simulink library "component_lib"  (R2023a)
settings: Solver=VariableStepAuto  StartTime=0.0  StopTime=10.0  RelTol=1e-3
undefined symbols (not defined in the file or in its folder): ECCV_r, par, R1234yf_ph, V_nom
libraries: base_lib x258, $bdroot x212, simulink x2, slpidlib x1
(part 1 of 7)
settings Model: Creator=maxjo65  LastModifiedBy=maxjo
settings SolverCC: AlgebraicLoopSolver=TrustRegion
settings OptimizationCC: ReuseModelBlockBuffer=off
settings DebuggingCC: UnconnectedInputMsg=warning  UnconnectedOutputMsg=warning  UnconnectedLineMsg=warning
settings ModelReferenceCC: EnableRefExpFcnMdlSchedulingChecks=on
settings RTWCC: DLArmComputeVersion=19.05

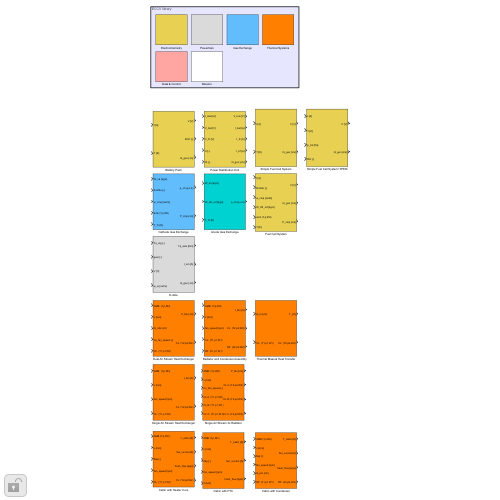
[thumbnail: Simulink's stored preview of the top-level diagram]
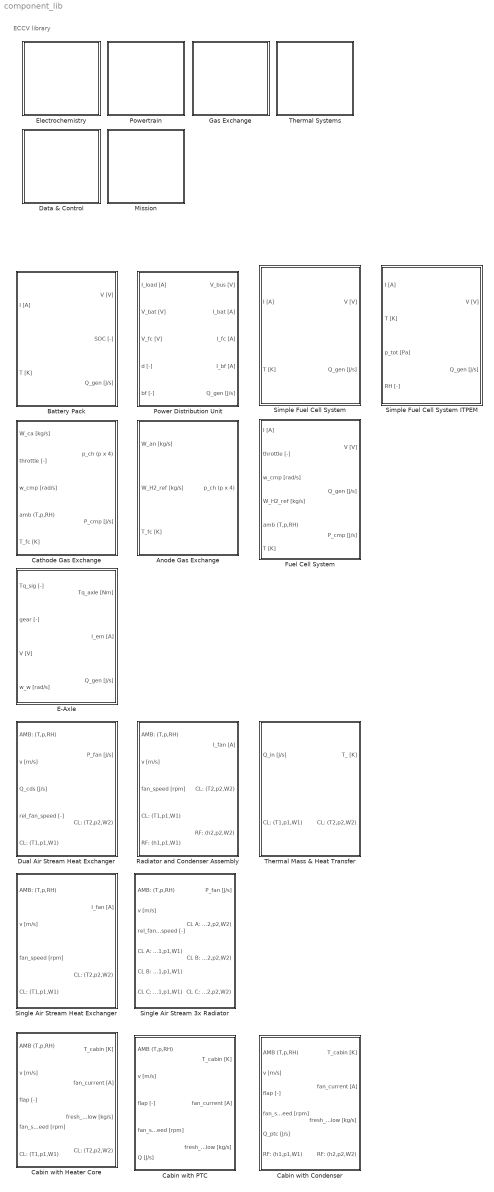
== system component_lib ==
  note: ECCV library
  Anode Gas Exchange : Subsystem
  Battery Pack : Subsystem  mask{SOC_0=0.5, Nx=74, Ny=6*16}
      mask prompts: SOC_0 "Initial charge [-]:"; Nx "Cells in parallel  [-]:"; Ny "Cells in series [-]:"
      mask init:
      | % parameter struct
      | par = struct;
      | 
      | % Get user-defined parameters
      | par.Ny = eval(get_param(gcb, 'Ny'));
      | par.Nx = eval(get_param(gcb, 'Nx'));
  Cabin with Condenser : Subsystem
  Cabin with Heater Core : Subsystem
  Cabin with PTC : Subsystem
  Cathode Gas Exchange : Subsystem
  Data & Control : Subsystem
  Dual Air Stream Heat Exchanger : Subsystem  mask{HtH=1.1, StS=0.95}
      mask prompts: HtH "Header to header [m]"; StS "Sideplate to sideplate [m]"
  E-Axle : Subsystem  mask{n=3, V_nom=700}
      mask prompts: n "Nr. of motors [-]"; V_nom "Nomnal voltage [V]:"
  Electrochemistry : Subsystem
  Fuel Cell System : Subsystem  mask{n_st=2, n=375}
      mask prompts: n_st "Stacks in series [#]:"; n "Cells per stack [#]:"
  Gas Exchange : Subsystem
  Mission : Subsystem
  Power Distribution Unit : Subsystem  mask{R_bf=1}
      mask prompts: R_bf "Burn-off resistance [Ohm]:"
  Powertrain : Subsystem
  Radiator and Condenser Assembly : Subsystem
  Simple Fuel Cell System : Subsystem  mask{n_st=2, n=375}
      mask prompts: n_st "Stacks in series [#]:"; n "Cells per stack [#]:"
  Simple Fuel Cell System ITPEM : Subsystem  mask{n_st=2, n=375, A_fc=400}
      mask prompts: n_st "Stacks in series [#]:"; n "Cells per stack [#]:"; A_fc "Membrane area [cm2]:"
  Single Air Stream 3x Radiator : Subsystem  mask{HtH=1.1, StS=0.95}
      mask prompts: HtH "Header to header [m]"; StS "Sideplate to sideplate [m]"
  Single Air Stream Heat Exchanger : Subsystem  mask{HtH=1.1, StS=0.95}
      mask prompts: HtH "Header to header [m]"; StS "Sideplate to sideplate [m]"
  Thermal Mass & Heat Transfer : Subsystem  mask{n=5, d=2e-3, L=50e-2, m=150, cp=420, T_0=273 + 20}
      mask prompts: n "Channels [-]:"; d "Hydraulic diameter [m]:"; L "Length [m]:"; m "Mass [kg]:"; cp "Heat capacity [J/kgK]:"; T_0 "Initial temperature [K]:"
  Thermal Systems : Subsystem

== system component_lib/Anode Gas Exchange ==
  W_an [kg/s] : Inport
  W_H2_ref [kg/s] : Inport  Port=2
  T_fc [K] : Inport  Port=3
  Channel Volume : $bdroot/Gas Exchange/GE0009_controlVolume  V=5e-3  p0=2.5e5  x0_H2=1  x0_O2=0  RH0=0.5
  GE0008_gasProperties : $bdroot/Gas Exchange/GE0008_gasProperties  SystemSampleTime=-1  VariantActivationTime=update diagram  Latency=0  AutoFrameSizeCalculation=off
  GE0008_gasProperties1 : $bdroot/Gas Exchange/GE0008_gasProperties  SystemSampleTime=-1  VariantActivationTime=update diagram  Latency=0  AutoFrameSizeCalculation=off
  GE0008_gasProperties2 : $bdroot/Gas Exchange/GE0008_gasProperties  SystemSampleTime=-1  VariantActivationTime=update diagram  Latency=0  AutoFrameSizeCalculation=off
  GE0013_ejector : $bdroot/Gas Exchange/GE0013_ejector  C_d=1  D_t=1.84e-3  Pi_lin=0.97  c_0=0.78406  c_1=-0.85801
  Hydrogen tank : $bdroot/Gas Exchange/GE0007_hydrogenTank  V=200e-3  T_tank=300  p_out=1.2e5  init_SOC=0.9  m0=5
  Linear Restriction : $bdroot/Gas Exchange/GE0015_linearRestriction  C_d=1e-5
  Linear Restriction1 : $bdroot/Gas Exchange/GE0015_linearRestriction  C_d=1e-5
  Primary manifold : $bdroot/Gas Exchange/GE0009_controlVolume  V=10e-3  p0=5e5  x0_H2=1  x0_O2=0  RH0=0.5
  Return Volume : $bdroot/Gas Exchange/GE0009_controlVolume  V=20e-3  p0=2.5e5  x0_H2=1  x0_O2=0  RH0=0.5
  SC0002_signalRead1 : $bdroot/Data & Control/SC0002_signalRead  SigName=anodeChannelPartialPressure
  SC0002_signalRead10 : $bdroot/Data & Control/SC0002_signalRead  SigName=anodeSupplyPartialPressure
  SC0002_signalRead11 : $bdroot/Data & Control/SC0002_signalRead  SigName=anodeChannelPressure
  SC0002_signalRead12 : $bdroot/Data & Control/SC0002_signalRead  SigName=anodeChannelHumidity
  SC0002_signalRead2 : $bdroot/Data & Control/SC0002_signalRead  SigName=anodeSupplyPressure
  SC0002_signalRead3 : $bdroot/Data & Control/SC0002_signalRead  SigName=anodeReturnPartialPressure
  SC0002_signalRead4 : $bdroot/Data & Control/SC0002_signalRead  SigName=entrainment
  SC0002_signalRead5 : $bdroot/Data & Control/SC0002_signalRead  SigName=recirculation
  SC0002_signalRead6 : $bdroot/Data & Control/SC0002_signalRead  SigName=anodePrimaryPressure
  SC0002_signalRead7 : $bdroot/Data & Control/SC0002_signalRead  SigName=anodeReturnPressure
  SC0002_signalRead8 : $bdroot/Data & Control/SC0002_signalRead  SigName=anodeReturnHumidity
  SC0002_signalRead9 : $bdroot/Data & Control/SC0002_signalRead  SigName=anodeSupplyHumidity
  Subsystem1 : Subsystem
      mask Display: disp('Anode Flow Stoichiometry Calculation');
  Sum : Sum  Inputs=+|+
  Sum1 : Sum  Inputs=|+-
  Sum2 : Sum  Inputs=+--
  Sum3 : Sum  Inputs=++-
  Sum5 : Sum  Inputs=1
  Sum8 : Sum  Inputs=-+|
  Supply Volume : $bdroot/Gas Exchange/GE0009_controlVolume  V=20e-3  p0=3e5  x0_H2=1  x0_O2=0  RH0=0.5
  p_ch (p x 4) : Outport
  wires:
  Sum1/1 -> Supply Volume/1
  GE0013_ejector/1 -> Sum/1, Sum8/1
  T_fc [K]/1 -> [T_fc], Channel Volume/2
  GE0013_ejector/4 -> SC0002_signalRead4/1
  GE0013_ejector/3 -> SC0002_signalRead5/1
  Hydrogen tank/2 -> Primary manifold/2, GE0013_ejector/2
  Sum8/1 -> Primary manifold/1
  Hydrogen tank/1 -> Sum8/2
  W_H2_ref [kg/s]/1 -> Hydrogen tank/1
  Sum5/1 -> SC0002_signalRead6/1
  Primary manifold/1 -> GE0013_ejector/1, Sum5/1
  GE0008_gasProperties/1 -> SC0002_signalRead2/1
  GE0013_ejector/2 -> Sum/2, Sum2/2
  Sum/1 -> Subsystem1/1(W_an), Sum1/1
  GE0008_gasProperties1/2 -> SC0002_signalRead8/1
  GE0008_gasProperties1/1 -> SC0002_signalRead7/1
  Linear Restriction/1 -> Sum3/3, Sum2/1
  Sum2/1 -> Return Volume/1
  Supply Volume/1 -> GE0013_ejector/5, Linear Restriction1/1, SC0002_signalRead10/1, GE0008_gasProperties/1
  Return Volume/1 -> SC0002_signalRead3/1, Linear Restriction/2, GE0013_ejector/3, GE0008_gasProperties1/1
  Sum3/1 -> Channel Volume/1
  Linear Restriction1/1 -> Sum1/2, Sum3/1
  W_an [kg/s]/1 -> Subsystem1/2(W_an_reacted), Sum3/2
  [T_fc] -> GE0013_ejector/4
  [T_fc] -> Return Volume/2
  [T_fc] -> GE0008_gasProperties1/2
  [T_fc] -> Supply Volume/2
  [T_fc] -> GE0008_gasProperties/2
  GE0008_gasProperties2/2 -> SC0002_signalRead12/1
  [T_fc] -> GE0008_gasProperties2/2
  Channel Volume/1 -> Linear Restriction/1, p_ch (p x 4)/1, GE0008_gasProperties2/1, SC0002_signalRead1/1, Linear Restriction1/2
  GE0008_gasProperties/2 -> SC0002_signalRead9/1
  GE0008_gasProperties2/1 -> SC0002_signalRead11/1

== system component_lib/Battery Pack ==
  I [A] : Inport
  T [K] : Inport  Port=2
  Battery current : $bdroot/Data & Control/SC0002_signalRead  SigName=batteryCurrent
  Cell current : $bdroot/Data & Control/SC0002_signalRead  SigName=batteryCellCurrent
  Cell voltage : $bdroot/Data & Control/SC0002_signalRead  SigName=batteryCellVoltage
  Constant1 : Constant  Value=Nx
  Constant2 : Constant  Value=Ny
  Constant4 : Constant  Value=Ny
  Constant5 : Constant  Value=Nx
  Divide : Product  Inputs=*/
  EL0001_panasonicNCR18650PF : $bdroot/Electrochemistry/EL0001_panasonicNCR18650PF  init_SOC=SOC_0
  Module voltage : $bdroot/Data & Control/SC0002_signalRead  SigName=batteryVoltage
  Module voltage1 : $bdroot/Data & Control/SC0002_signalRead  SigName=batteryPower
  Product1 : Product
  Product2 : Product  Inputs=3
  Product3 : Product
  SOC : $bdroot/Data & Control/SC0002_signalRead  SigName=stateOfCharge
  V [V] : Outport
  SOC [-] : Outport  Port=2
  Q_gen [J/s] : Outport  Port=3
  wires:
  Product1/1 -> Product3/2, Module voltage/1, V [V]/1
  EL0001_panasonicNCR18650PF/2 -> SOC/1, SOC [-]/1
  Constant2/1 -> Product1/1
  EL0001_panasonicNCR18650PF/1 -> Cell voltage/1, Product1/2
  Divide/1 -> EL0001_panasonicNCR18650PF/1, Cell current/1
  I [A]/1 -> Product3/1, Battery current/1, Divide/1
  Constant1/1 -> Divide/2
  T [K]/1 -> EL0001_panasonicNCR18650PF/2
  EL0001_panasonicNCR18650PF/3 -> Product2/1
  Constant5/1 -> Product2/3
  Constant4/1 -> Product2/2
  Product2/1 -> Q_gen [J/s]/1
  Product3/1 -> Module voltage1/1

== system component_lib/Cabin with Condenser ==
  AMB (T,p,RH) : Inport
  v [m/s] : Inport  Port=2
  flap [-] : Inport  Port=3
  fan_speed [rpm] : Inport  Port=4
  Q_ptc [J/s] : Inport  Port=5
  RF: (h1,p1,W1) : Inport  Port=6
  Add Constant : Bias  Bias=-273.15  SaturateOnIntegerOverflow=off
  Cabin Air Volume : $bdroot/Thermal Systems/TH0026_airVolume  V=4  T0=273.15 + 20
  Constant : Constant  Value=24
  Constant6 : Constant
  Demux : Demux  Outputs=3
  Demux1 : Demux  Outputs=3
  Intake Flap : $bdroot/Thermal Systems/TH0027_hvacFlap  A=0.04  zeta=0.3
  Mux : Mux  Inputs=3
  RF0013_calculateHeatflow : $bdroot/Thermal Systems/RF0013_calculateHeatflow
  RF0020_simpleLouverFinHEX : $bdroot/Thermal Systems/RF0020_simpleLouverFinHEX  N_tub=60  T_L=0.95*3  T_p=10.15e-3  T_d=16e-3  N_ch=18  a=1.3e-3  b=0.58e-3  L_a=23  F_p=1.4e-3  L_p=1.7e-3  L_l=6.4e-3  H=8.15e-3  d_f=16e-3  F_d=16e-3
  SC0002_signalRead1 : $bdroot/Data & Control/SC0002_signalRead  SigName=cabinTemperature
  SC0002_signalRead6 : $bdroot/Data & Control/SC0002_signalRead  SigName=cabinHeating
  SC0002_signalRead8 : $bdroot/Data & Control/SC0002_signalRead  SigName=cabinConvection
  TH0005_flowSplit : $bdroot/Thermal Systems/TH0005_flowSplit  SystemSampleTime=-1  VariantActivationTime=update diagram  Latency=0  AutoFrameSizeCalculation=off
  TH0006_flowConfluence : $bdroot/Thermal Systems/TH0006_flowConfluence  gain=0.01
  TH0009_intake : $bdroot/Thermal Systems/TH0009_intake  zeta=0.1
  TH0011_outletFlowBalance : $bdroot/Thermal Systems/TH0011_outletFlowBalance  gain=0.05
  TH0019_airTotalHeatTransfer : $bdroot/Thermal Systems/TH0019_airTotalHeatTransfer  T_min=273-40  T_max=273+140
  TH0028_VA195 : $bdroot/Thermal Systems/TH0028_VA195  n=4
      settings: LibrarySourceBlock=component_lib/Thermal Systems/TH0023_WP120
  TH0029_cabinConvection : $bdroot/Thermal Systems/TH0029_cabinConvection  A=2
  Terminator : Terminator
  Terminator1 : Terminator
  Terminator2 : Terminator
  outletFlap : $bdroot/Thermal Systems/TH0027_hvacFlap  A=0.04  zeta=0.3
  T_cabin [K] : Outport
  fan_current [A] : Outport  Port=2
  fresh_flow [kg/s] : Outport  Port=3
  RF: (h2,p2,W2) : Outport  Port=4
  wires:
  Demux/3 -> fresh_flow [kg/s]/1
  [p_amb] -> TH0011_outletFlowBalance/2
  Constant6/1 -> outletFlap/1
  TH0011_outletFlowBalance/1 -> [W_in]
  [W_in] -> Mux/3
  RF0020_simpleLouverFinHEX/1 -> RF: (h2,p2,W2)/1, RF0013_calculateHeatflow/1
  Demux1/1 -> Mux/1, [T_amb]
  outletFlap/1 -> TH0011_outletFlowBalance/1
  Demux1/2 -> Mux/2, [p_amb]
  RF: (h1,p1,W1)/1 -> RF0020_simpleLouverFinHEX/1, RF0013_calculateHeatflow/2
  RF0013_calculateHeatflow/1 -> SC0002_signalRead6/1
  Mux/1 -> TH0009_intake/1, Demux/1
  TH0005_flowSplit/1 -> TH0028_VA195/3
  TH0029_cabinConvection/1 -> Cabin Air Volume/1, SC0002_signalRead8/1
  TH0006_flowConfluence/2 -> TH0005_flowSplit/2
  TH0005_flowSplit/2 -> outletFlap/2
  Cabin Air Volume/1 -> TH0029_cabinConvection/3, Add Constant/1, T_cabin [K]/1
  [v] -> TH0029_cabinConvection/1
  v [m/s]/1 -> [v], TH0009_intake/2
  TH0028_VA195/1 -> fan_current [A]/1
  [T_amb] -> TH0029_cabinConvection/2
  Intake Flap/1 -> TH0006_flowConfluence/2
  fan_speed [rpm]/1 -> TH0028_VA195/2
  Constant/1 -> TH0028_VA195/1
  flap [-]/1 -> Intake Flap/1
  AMB (T,p,RH)/1 -> Demux1/1
  Cabin Air Volume/2 -> TH0005_flowSplit/1
  TH0009_intake/1 -> Intake Flap/2
  Demux/1 -> Terminator/1
  Demux/2 -> Terminator1/1
  Demux1/3 -> Terminator2/1
  Add Constant/1 -> SC0002_signalRead1/1
  Q_ptc [J/s]/1 -> TH0019_airTotalHeatTransfer/1
  TH0006_flowConfluence/1 -> RF0020_simpleLouverFinHEX/2
  TH0028_VA195/2 -> TH0006_flowConfluence/1
  RF0020_simpleLouverFinHEX/2 -> TH0019_airTotalHeatTransfer/2
  TH0019_airTotalHeatTransfer/1 -> Cabin Air Volume/2

== system component_lib/Cabin with Heater Core ==
  AMB (T,p,RH) : Inport
  v [m/s] : Inport  Port=2
  flap [-] : Inport  Port=3
  fan_speed [rpm] : Inport  Port=4
  CL: (T1,p1,W1) : Inport  Port=5
  Add Constant : Bias  Bias=-273.15  SaturateOnIntegerOverflow=off
  Cabin Air Volume : $bdroot/Thermal Systems/TH0026_airVolume  V=4  T0=273.15 + 20
  Constant : Constant  Value=24
  Constant6 : Constant
  Demux : Demux  Outputs=3
  Demux1 : Demux  Outputs=3
  Heat Exchanger : $bdroot/Thermal Systems/TH0002_radiatorCore  HtH=0.4  StS=0.4  radmodel=24 mm
  Intake Flap : $bdroot/Thermal Systems/TH0027_hvacFlap  A=0.04  zeta=0.3
  Mux : Mux  Inputs=3
  SC0002_signalRead1 : $bdroot/Data & Control/SC0002_signalRead  SigName=cabinTemperature
  SC0002_signalRead6 : $bdroot/Data & Control/SC0002_signalRead  SigName=cabinHeating
  SC0002_signalRead8 : $bdroot/Data & Control/SC0002_signalRead  SigName=cabinConvection
  TH0005_flowSplit : $bdroot/Thermal Systems/TH0005_flowSplit  SystemSampleTime=-1  VariantActivationTime=update diagram  Latency=0  AutoFrameSizeCalculation=off
  TH0006_flowConfluence : $bdroot/Thermal Systems/TH0006_flowConfluence  gain=0.01
  TH0009_intake : $bdroot/Thermal Systems/TH0009_intake  zeta=0.1
  TH0011_outletFlowBalance : $bdroot/Thermal Systems/TH0011_outletFlowBalance  gain=0.05
  TH0028_VA195 : $bdroot/Thermal Systems/TH0028_VA195  n=1
      settings: LibrarySourceBlock=component_lib/Thermal Systems/TH0023_WP120
  TH0029_cabinConvection : $bdroot/Thermal Systems/TH0029_cabinConvection  A=5
  Terminator : Terminator
  Terminator1 : Terminator
  Terminator2 : Terminator
  outletFlap : $bdroot/Thermal Systems/TH0027_hvacFlap  A=0.04  zeta=0.3
  T_cabin [K] : Outport
  fan_current [A] : Outport  Port=2
  fresh_flow [kg/s] : Outport  Port=3
  CL: (T2,p2,W2) : Outport  Port=4
  wires:
  Demux/3 -> fresh_flow [kg/s]/1
  [p_amb] -> TH0011_outletFlowBalance/2
  Constant6/1 -> outletFlap/1
  TH0011_outletFlowBalance/1 -> [W_in]
  [W_in] -> Mux/3
  Heat Exchanger/3 -> CL: (T2,p2,W2)/1
  Demux1/1 -> Mux/1, [T_amb]
  outletFlap/1 -> TH0011_outletFlowBalance/1
  Demux1/2 -> Mux/2, [p_amb]
  CL: (T1,p1,W1)/1 -> Heat Exchanger/2
  Heat Exchanger/1 -> SC0002_signalRead6/1
  Mux/1 -> Demux/1, TH0009_intake/1
  TH0005_flowSplit/1 -> TH0028_VA195/3
  TH0029_cabinConvection/1 -> Cabin Air Volume/1, SC0002_signalRead8/1
  TH0006_flowConfluence/2 -> TH0005_flowSplit/2
  TH0005_flowSplit/2 -> outletFlap/2
  Cabin Air Volume/1 -> TH0029_cabinConvection/3, Add Constant/1, T_cabin [K]/1
  [v] -> TH0029_cabinConvection/1
  Heat Exchanger/2 -> Cabin Air Volume/2
  v [m/s]/1 -> [v], TH0009_intake/2
  TH0028_VA195/1 -> fan_current [A]/1
  [T_amb] -> TH0029_cabinConvection/2
  Intake Flap/1 -> TH0006_flowConfluence/2
  fan_speed [rpm]/1 -> TH0028_VA195/2
  Constant/1 -> TH0028_VA195/1
  flap [-]/1 -> Intake Flap/1
  AMB (T,p,RH)/1 -> Demux1/1
  Cabin Air Volume/2 -> TH0005_flowSplit/1
  TH0006_flowConfluence/1 -> Heat Exchanger/1
  TH0009_intake/1 -> Intake Flap/2
  TH0028_VA195/2 -> TH0006_flowConfluence/1
  Demux/1 -> Terminator/1
  Demux/2 -> Terminator1/1
  Demux1/3 -> Terminator2/1
  Add Constant/1 -> SC0002_signalRead1/1

== system component_lib/Cabin with PTC ==
  AMB (T,p,RH) : Inport
  v [m/s] : Inport  Port=2
  flap [-] : Inport  Port=3
  fan_speed [rpm] : Inport  Port=4
  Q [J/s] : Inport  Port=5
  Add Constant : Bias  Bias=-273.15  SaturateOnIntegerOverflow=off
  Cabin Air Volume : $bdroot/Thermal Systems/TH0026_airVolume  V=4  T0=273.15 + 20
  Constant4 : Constant  Value=24
  Constant6 : Constant
  Demux : Demux  Outputs=3
  Demux1 : Demux  Outputs=3
  Intake Flap : $bdroot/Thermal Systems/TH0027_hvacFlap  A=0.04  zeta=0.3
  Mux : Mux  Inputs=3
  SC0002_signalRead1 : $bdroot/Data & Control/SC0002_signalRead  SigName=cabinTemperature
  SC0002_signalRead6 : $bdroot/Data & Control/SC0002_signalRead  SigName=cabinHeating
  SC0002_signalRead8 : $bdroot/Data & Control/SC0002_signalRead  SigName=cabinConvection
  TH0005_flowSplit : $bdroot/Thermal Systems/TH0005_flowSplit  SystemSampleTime=-1  VariantActivationTime=update diagram  Latency=0  AutoFrameSizeCalculation=off
  TH0006_flowConfluence : $bdroot/Thermal Systems/TH0006_flowConfluence  gain=0.01
  TH0009_intake : $bdroot/Thermal Systems/TH0009_intake  zeta=0.1
  TH0011_outletFlowBalance : $bdroot/Thermal Systems/TH0011_outletFlowBalance  gain=0.05
  TH0019_airTotalHeatTransfer : $bdroot/Thermal Systems/TH0019_airTotalHeatTransfer  T_min=273-40  T_max=273+140
  TH0028_VA195 : $bdroot/Thermal Systems/TH0028_VA195  n=1
      settings: LibrarySourceBlock=component_lib/Thermal Systems/TH0023_WP120
  TH0029_cabinConvection : $bdroot/Thermal Systems/TH0029_cabinConvection  A=5
  Terminator : Terminator
  Terminator1 : Terminator
  Terminator2 : Terminator
  outletFlap : $bdroot/Thermal Systems/TH0027_hvacFlap  A=0.04  zeta=0.3
  T_cabin [K] : Outport
  fan_current [A] : Outport  Port=2
  fresh_flow [kg/s] : Outport  Port=3
  wires:
  Demux/3 -> fresh_flow [kg/s]/1
  [p_amb] -> TH0011_outletFlowBalance/2
  Constant6/1 -> outletFlap/1
  TH0011_outletFlowBalance/1 -> [W_in]
  [W_in] -> Mux/3
  Demux1/1 -> Mux/1, [T_amb]
  outletFlap/1 -> TH0011_outletFlowBalance/1
  Demux1/2 -> Mux/2, [p_amb]
  Q [J/s]/1 -> SC0002_signalRead6/1, TH0019_airTotalHeatTransfer/1
  Mux/1 -> Demux/1, TH0009_intake/1
  TH0005_flowSplit/1 -> TH0028_VA195/3
  TH0029_cabinConvection/1 -> Cabin Air Volume/1, SC0002_signalRead8/1
  TH0006_flowConfluence/2 -> TH0005_flowSplit/2
  TH0005_flowSplit/2 -> outletFlap/2
  Cabin Air Volume/1 -> TH0029_cabinConvection/3, Add Constant/1, T_cabin [K]/1
  [v] -> TH0029_cabinConvection/1
  TH0019_airTotalHeatTransfer/1 -> Cabin Air Volume/2
  v [m/s]/1 -> [v], TH0009_intake/2
  TH0028_VA195/1 -> fan_current [A]/1
  [T_amb] -> TH0029_cabinConvection/2
  Intake Flap/1 -> TH0006_flowConfluence/2
  fan_speed [rpm]/1 -> TH0028_VA195/2
  Constant4/1 -> TH0028_VA195/1
  flap [-]/1 -> Intake Flap/1
  AMB (T,p,RH)/1 -> Demux1/1
  Cabin Air Volume/2 -> TH0005_flowSplit/1
  TH0009_intake/1 -> Intake Flap/2
  TH0028_VA195/2 -> TH0006_flowConfluence/1
  Demux/1 -> Terminator/1
  Demux/2 -> Terminator1/1
  Demux1/3 -> Terminator2/1
  Add Constant/1 -> SC0002_signalRead1/1
  TH0006_flowConfluence/1 -> TH0019_airTotalHeatTransfer/2

== system component_lib/Cathode Gas Exchange ==
  note: Compressor Dynamics
  W_ca [kg/s] : Inport
  throttle [-] : Inport  Port=2
  w_cmp [rad/s] : Inport  Port=3
  amb (T,p,RH) : Inport  Port=4
  T_fc [K] : Inport  Port=5
  Channel Volume : $bdroot/Gas Exchange/GE0009_controlVolume  V=10e-3  p0=2.3e5  x0_H2=0  x0_O2=0.21  RH0=0.8
  Demux : Demux  Outputs=3
  Demux1 : Demux  Outputs=3
  GE0002_dynHumidGasSupply : $bdroot/Gas Exchange/GE0002_dynHumidGasSupply  x_H2_dry=0  x_O2_dry=0.21
  GE0002_dynHumidGasSupply1 : $bdroot/Gas Exchange/GE0002_dynHumidGasSupply  x_H2_dry=0  x_O2_dry=0.21
  GE0008_gasProperties : $bdroot/Gas Exchange/GE0008_gasProperties  SystemSampleTime=-1  VariantActivationTime=update diagram  Latency=0  AutoFrameSizeCalculation=off
  GE0008_gasProperties1 : $bdroot/Gas Exchange/GE0008_gasProperties  SystemSampleTime=-1  VariantActivationTime=update diagram  Latency=0  AutoFrameSizeCalculation=off
  GE0008_gasProperties2 : $bdroot/Gas Exchange/GE0008_gasProperties  SystemSampleTime=-1  VariantActivationTime=update diagram  Latency=0  AutoFrameSizeCalculation=off
  GE0011_ellipseCompressor : $bdroot/Gas Exchange/GE0011_ellipseCompressor  compressor_parameters=param_TD04.mat  w0=15e3
  GE0012_throttle : $bdroot/Gas Exchange/GE0012_throttle  a0=1.3229e-05  a1=9.4736e-05  a2=0.0029  Pi_lin=0.97
  GE0015_linearRestriction : $bdroot/Gas Exchange/GE0015_linearRestriction  C_d=1e-5
  GE0015_linearRestriction1 : $bdroot/Gas Exchange/GE0015_linearRestriction  C_d=1e-5
  Gain : Gain
  Integrator Limited : Integrator  InitialCondition=1e4  LimitOutput=on  UpperSaturationLimit=2e4  LowerSaturationLimit=3e3
  Return Volume : $bdroot/Gas Exchange/GE0009_controlVolume  V=40e-3  p0=2e5  x0_H2=0  x0_O2=0.21  RH0=0.8
  SC0002_signalRead1 : $bdroot/Data & Control/SC0002_signalRead  SigName=compressorFlow
  SC0002_signalRead10 : $bdroot/Data & Control/SC0002_signalRead  SigName=cathodeReturnPressure
  SC0002_signalRead11 : $bdroot/Data & Control/SC0002_signalRead  SigName=cathodeReturnHumidity
  SC0002_signalRead12 : $bdroot/Data & Control/SC0002_signalRead  SigName=cathodeReturnPartialPressure
  SC0002_signalRead2 : $bdroot/Data & Control/SC0002_signalRead  SigName=throttlePosition
  SC0002_signalRead3 : $bdroot/Data & Control/SC0002_signalRead  SigName=cathodeSupplyPartialPressure
  SC0002_signalRead4 : $bdroot/Data & Control/SC0002_signalRead  SigName=compressorSpeed
  SC0002_signalRead5 : $bdroot/Data & Control/SC0002_signalRead  SigName=cathodeSupplyPressure
  SC0002_signalRead6 : $bdroot/Data & Control/SC0002_signalRead  SigName=cathodeChannelPressure
  SC0002_signalRead7 : $bdroot/Data & Control/SC0002_signalRead  SigName=cathodeChannelHumidity
  SC0002_signalRead8 : $bdroot/Data & Control/SC0002_signalRead  SigName=cathodeChannelPartialPressure
  SC0002_signalRead9 : $bdroot/Data & Control/SC0002_signalRead  SigName=cathodeSupplyHumidity
  Subsystem1 : Subsystem
      mask Display: disp('Cathode Flow Stoichiometry Calculation');
  Sum : Sum  Inputs=|+-
  Sum1 : Sum  Inputs=1
  Sum2 : Sum  Inputs=|+-
  Sum3 : Sum  Inputs=+-|
  Sum4 : Sum  Inputs=++-
  Supply Volume : $bdroot/Gas Exchange/GE0009_controlVolume  V=40e-3  p0=2.5e5  x0_H2=0  x0_O2=0.21  RH0=0.8
  Terminator : Terminator
  Terminator1 : Terminator
  p_ch (p x 4) : Outport
  P_cmp [J/s] : Outport  Port=2
  wires:
  Sum1/1 -> SC0002_signalRead1/1
  Gain/1 -> Integrator Limited/1
  Integrator Limited/1 -> SC0002_signalRead4/1, GE0011_ellipseCompressor/4, Sum/2
  Sum/1 -> Gain/1
  w_cmp [rad/s]/1 -> Sum/1
  GE0002_dynHumidGasSupply/1 -> GE0011_ellipseCompressor/1
  GE0002_dynHumidGasSupply1/1 -> GE0012_throttle/3
  GE0002_dynHumidGasSupply/2 -> GE0011_ellipseCompressor/2
  GE0011_ellipseCompressor/1 -> Sum2/1, Sum1/1, Subsystem1/1(W_ca)
  throttle [-]/1 -> SC0002_signalRead2/1, GE0012_throttle/4
  Demux/1 -> GE0002_dynHumidGasSupply/1
  Demux/2 -> GE0002_dynHumidGasSupply/2
  Demux/3 -> GE0002_dynHumidGasSupply/3
  Demux1/1 -> GE0002_dynHumidGasSupply1/1
  Demux1/2 -> GE0002_dynHumidGasSupply1/2
  Demux1/3 -> GE0002_dynHumidGasSupply1/3
  amb (T,p,RH)/1 -> Demux/1, Demux1/1
  GE0008_gasProperties/1 -> SC0002_signalRead5/1
  Supply Volume/1 -> GE0015_linearRestriction1/1, GE0008_gasProperties/1, GE0011_ellipseCompressor/3, SC0002_signalRead3/1
  GE0008_gasProperties/2 -> SC0002_signalRead9/1
  Sum2/1 -> Supply Volume/1
  GE0011_ellipseCompressor/3 -> P_cmp [J/s]/1
  GE0015_linearRestriction/1 -> Sum4/3, Sum3/1
  T_fc [K]/1 -> [T_fc], Supply Volume/2
  Sum3/1 -> Return Volume/1
  GE0012_throttle/1 -> Sum3/2
  GE0012_throttle/2 -> Terminator/1
  GE0011_ellipseCompressor/2 -> Terminator1/1
  [T_fc] -> Return Volume/2
  [T_fc] -> GE0008_gasProperties/2
  [T_fc] -> GE0012_throttle/2
  Channel Volume/1 -> p_ch (p x 4)/1, GE0015_linearRestriction/1, GE0008_gasProperties1/1, GE0015_linearRestriction1/2, SC0002_signalRead8/1
  W_ca [kg/s]/1 -> Sum4/2, Subsystem1/2(W_ca_reacted)
  GE0015_linearRestriction1/1 -> Sum4/1, Sum2/2
  Sum4/1 -> Channel Volume/1
  [T_fc] -> Channel Volume/2
  [T_fc] -> GE0008_gasProperties1/2
  GE0008_gasProperties1/1 -> SC0002_signalRead6/1
  GE0008_gasProperties1/2 -> SC0002_signalRead7/1
  GE0008_gasProperties2/1 -> SC0002_signalRead10/1
  GE0008_gasProperties2/2 -> SC0002_signalRead11/1
  [T_fc] -> GE0008_gasProperties2/2
  Return Volume/1 -> GE0008_gasProperties2/1, GE0012_throttle/1, GE0015_linearRestriction/2, SC0002_signalRead12/1

== system component_lib/Data & Control ==
  DC0007_cathodeFlowControl : Subsystem  mask{lambda_O2_ref=2, n_cell=455}
      mask prompts: lambda_O2_ref "Oxygen stoich. reference [-]:"; n_cell "Nr. of cells [-]:"
  DC0008_linearMPCSolver : Subsystem  mask{N=1, Q=1, R=1, n_A=1, m_B=1}
      mask prompts: N "Prediction horizon (N):"; Q "Q-matrix:"; R "R-matrix:"; n_A "Rows in A (n):"; m_B "Columns in B (m):"
      mask DialogControl Container3 Prompt: Matrix Sizes:
  SC0002_signalRead : Subsystem  mask{SigName=SigIdentifier}
      mask prompts: SigName "Signal identifier:"
      mask init:
      | % set name of input port
      | blockNames = Simulink.findBlocks(gcb);
      | set(blockNames(1), 'Name', SigName);
      | 
      | % log input port
      | ph = get_param([gcb, '/', SigName], 'PortHandles');
      | set_param(ph.Outport(1), 'DataLogging', 'on')
      | 
      | % set signal name in goto tag
      | set_param([gcb, '/', 'Goto'], 'GotoTag', SigName)
      mask Display: disp(SigName)
  SC0003_signalWrite : Subsystem  mask{SigName=SigIdentifier}
      mask prompts: SigName "Signal identifier:"
      mask init:
      | % set signal name in goto tag
      | set_param([gcb, '/', 'From'], 'GotoTag', SigName)
      mask Display: disp(SigName)

== system component_lib/Dual Air Stream Heat Exchanger ==
  AMB: (T,p,RH) : Inport
  v [m/s] : Inport  Port=2
  Q_cds [J/s] : Inport  Port=3
  rel_fan_speed [-] : Inport  Port=4
  CL: (T1,p1,W1) : Inport  Port=5
  Demux : Demux  Outputs=3
  Mux : Mux  Inputs=3
  Radiator core - behind CDS : $bdroot/Thermal Systems/TH0002_radiatorCore  HtH=0.35  StS=0.95  radmodel=52 mm
  Radiator core - exposed : $bdroot/Thermal Systems/TH0002_radiatorCore  HtH=1.1-0.35  StS=0.95  radmodel=52 mm
  TH0003_coolantTank : $bdroot/Thermal Systems/TH0003_coolantTank  StS=0.95  D_con=0.055  T_0=286  radmodel=52 mm
  TH0003_coolantTank1 : $bdroot/Thermal Systems/TH0003_coolantTank  StS=0.95  D_con=0.055  T_0=286  radmodel=52 mm
  TH0004_radiatorPlugFlow : $bdroot/Thermal Systems/TH0004_radiatorPlugFlow  HtH=1.1  StS=0.95  T_0=286  radmodel=52 mm
  TH0005_flowSplit : $bdroot/Thermal Systems/TH0005_flowSplit  SystemSampleTime=-1  VariantActivationTime=update diagram  Latency=0  AutoFrameSizeCalculation=off
  TH0006_flowConfluence : $bdroot/Thermal Systems/TH0006_flowConfluence  gain=0.01
  TH0007_airRestriction : $bdroot/Thermal Systems/TH0007_airRestriction  A=0.8  zeta=0.3
  TH0007_airRestriction1 : $bdroot/Thermal Systems/TH0007_airRestriction  A=1  zeta=2.5
  TH0008_condenser : $bdroot/Thermal Systems/TH0008_condenser  HtH=0.85  StS=0.35  cdsmodel=18.8 mm
  TH0009_intake : $bdroot/Thermal Systems/TH0009_intake  zeta=0.9
  TH0010_fan : $bdroot/Thermal Systems/TH0010_fan  n_fan=4
  TH0011_outletFlowBalance : $bdroot/Thermal Systems/TH0011_outletFlowBalance  gain=0.05
  P_fan [J/s] : Outport
  CL: (T2,p2,W2) : Outport  Port=2
  wires:
  Demux/2 -> Mux/2, [p_amb]
  Demux/1 -> Mux/1
  AMB: (T,p,RH)/1 -> Demux/1
  TH0003_coolantTank1/1 -> CL: (T2,p2,W2)/1
  TH0010_fan/2 -> P_fan [J/s]/1
  rel_fan_speed [-]/1 -> TH0010_fan/2
  TH0005_flowSplit/1 -> TH0008_condenser/1
  v [m/s]/1 -> TH0009_intake/2
  TH0007_airRestriction/1 -> TH0005_flowSplit/1
  TH0004_radiatorPlugFlow/1 -> TH0003_coolantTank1/1
  TH0007_airRestriction1/1 -> TH0011_outletFlowBalance/1
  TH0003_coolantTank/1 -> Radiator core - behind CDS/2
  Q_cds [J/s]/1 -> TH0008_condenser/2
  CL: (T1,p1,W1)/1 -> TH0003_coolantTank/1
  TH0006_flowConfluence/2 -> TH0005_flowSplit/2
  TH0006_flowConfluence/1 -> TH0010_fan/1
  Mux/1 -> TH0009_intake/1
  TH0005_flowSplit/2 -> [air_22]
  TH0009_intake/1 -> TH0007_airRestriction/1
  TH0008_condenser/1 -> Radiator core - behind CDS/1
  Radiator core - behind CDS/2 -> TH0006_flowConfluence/1
  Radiator core - exposed/2 -> TH0006_flowConfluence/2
  Radiator core - behind CDS/3 -> Radiator core - exposed/2
  [p_amb] -> TH0011_outletFlowBalance/2
  [air_22] -> Radiator core - exposed/1
  TH0010_fan/1 -> TH0007_airRestriction1/1
  Radiator core - exposed/3 -> TH0004_radiatorPlugFlow/1
  TH0011_outletFlowBalance/1 -> [W_in]
  [W_in] -> Mux/3

== system component_lib/E-Axle ==
  note: Input as % of max. torque at current speed
  Tq_sig [-] : Inport
  gear [-] : Inport  Port=2
  V [V] : Inport  Port=3
  w_w [rad/s] : Inport  Port=4
  Constant1 : Constant  Value=V_nom
  Constant3 : Constant
  Current sensor : $bdroot/Data & Control/SC0002_signalRead  SigName=motorCurrent
  Divide : Product  Inputs=**/
  Divide1 : Product  Inputs=**
  Gain : Gain  Gain=n
  Gain1 : Gain  Gain=n
  Gain2 : Gain  Gain=n
  Gain3 : Gain  Gain=-1
  Max torque : $bdroot/Data & Control/SC0002_signalRead  SigName=maxMotorTorque
  Min torque : $bdroot/Data & Control/SC0002_signalRead  SigName=minMotorTorque
  PT0002_simpleMotor : $bdroot/Powertrain/PT0002_simpleMotor  T_s=0.1
  PT0003_gearBox : $bdroot/Powertrain/PT0003_gearBox  fd_ratio=2  gear_ratios=[5 3.8 2.3 1.15]  eta_gb=0.98
  Saturation2 : Saturate  UpperLimit=1  LowerLimit=-1
  Saturation3 : Saturate  UpperLimit=476  LowerLimit=0
  Saturation4 : Saturate  UpperLimit=V_nom  LowerLimit=0
  Speed sensor : $bdroot/Data & Control/SC0002_signalRead  SigName=motorSpeed
  Torque sensor : $bdroot/Data & Control/SC0002_signalRead  SigName=motorTorque
  speed-Torque map1 : Lookup_n-D  NumberOfTableDimensions=1  BreakpointsForDimension1=|  Table=|  ExtrapMethod=Clip  UseLastTableValue=on  InternalRulePriority=Speed  RndMeth=Simplest
      BreakpointsForDimension1=|
      | [25.2590673575129
      | 34.9740932642487
      | 43.3937823834197
      | 51.1658031088083
      | 55.6994818652850
      | 64.1191709844560
      | 65.4145077720207
      | 67.3575129533679
      | 68.0051813471503
      | 69.9481865284974
      | 71.2435233160622
      | 73.1865284974093
      | 75.7772020725389
      | 76.4248704663213
      | 78.3678756476684
      | 81.6062176165803
      | 82.9015544041451
      | 86.1398963730570
      | 88.0829015544041
      | 90.0259067357513
      | 94.5595854922280
      | 97.1502590673575
      | 100.388601036269
      | 103.626943005181
      | 109.455958549223
      | 113.989637305699
      | 120.466321243523
      | 125.000000000000
      | 128.238341968912
      | 133.419689119171
      | 139.248704663212
      | 145.077720207254
      | 150.259067357513
      | 158.031088082902
      | 164.507772020725
      | 172.279792746114
      | 174.870466321244
      | 195.595854922280
      | 211.139896373057
      | 221.502590673575
      | 229.922279792746
      | 244.818652849741
      | 256.476683937824
      | 270.725388601036
      | 284.974093264249
      | 290.155440414508
      | 300.518134715026
      | 313.471502590674
      | 324.481865284974
      | 344.559585492228
      | 356.217616580311
      | 366.580310880829
      | 376.295336787565
      | 384.067357512953
      | 403.497409326425
      | 422.927461139896
      | 438.471502590674
      | 453.367875647669
      | 465.025906735751
      | 476.036269430052]
      Table=|
      | [1991.26637554585
      | 1997.08879184862
      | 1994.17758369723
      | 1994.17758369723
      | 1994.17758369723
      | 1991.26637554585
      | 1944.68704512373
      | 1921.39737991266
      | 1854.43959243086
      | 1816.59388646288
      | 1787.48180494905
      | 1700.14556040757
      | 1671.03347889374
      | 1621.54294032023
      | 1548.76273653566
      | 1513.82823871907
      | 1438.13682678311
      | 1391.55749636099
      | 1339.15574963610
      | 1280.93158660844
      | 1225.61863173217
      | 1176.12809315866
      | 1129.54876273654
      | 1085.88064046579
      | 1018.92285298399
      | 969.432314410480
      | 925.764192139738
      | 876.273653566230
      | 835.516739446870
      | 797.671033478894
      | 756.914119359534
      | 727.802037845706
      | 704.512372634643
      | 666.666666666667
      | 628.820960698690
      | 602.620087336244
      | 588.064046579330
      | 518.195050946142
      | 477.438136826783
      | 445.414847161572
      | 410.480349344978
      | 395.924308588064
      | 375.545851528384
      | 343.522561863173
      | 328.966521106259
      | 320.232896652110
      | 302.765647743814
      | 282.387190684134
      | 282.387190684134
      | 259.097525473071
      | 244.541484716157
      | 244.541484716157
      | 221.251819505094
      | 221.251819505094
      | 209.606986899563
      | 195.050946142649
      | 189.228529839883
      | 183.406113537118
      | 174.672489082969
      | 157.205240174672]
  Tq_axle [Nm] : Outport
  I_em [A] : Outport  Port=2
  Q_gen [J/s] : Outport  Port=3
  wires:
  Gain2/1 -> Tq_axle [Nm]/1
  PT0003_gearBox/1 -> Gain2/1
  PT0002_simpleMotor/3 -> Gain/1
  Gain1/1 -> Current sensor/1, I_em [A]/1
  PT0002_simpleMotor/1 -> PT0003_gearBox/1, Torque sensor/1
  Constant3/1 -> PT0003_gearBox/4
  gear [-]/1 -> PT0003_gearBox/3
  PT0003_gearBox/2 -> Divide/1, PT0002_simpleMotor/3, Speed sensor/1
  w_w [rad/s]/1 -> PT0003_gearBox/2
  PT0002_simpleMotor/2 -> Gain1/1
  Gain/1 -> Q_gen [J/s]/1
  Gain3/1 -> Min torque/1
  V [V]/1 -> PT0002_simpleMotor/2, Saturation4/1
  speed-Torque map1/1 -> Divide1/2, Gain3/1, Max torque/1
  Saturation2/1 -> Divide1/1
  Saturation4/1 -> Divide/3
  Saturation3/1 -> speed-Torque map1/1
  Divide1/1 -> PT0002_simpleMotor/1
  Tq_sig [-]/1 -> Saturation2/1
  Constant1/1 -> Divide/2
  Divide/1 -> Saturation3/1

== system component_lib/Electrochemistry ==
  EL0001_panasonicNCR18650PF : Subsystem  mask{init_SOC=0.2380}
      mask prompts: init_SOC "Initial SOC [-]:"
      mask init:
      | % parameter struct
      | par = struct;
      | 
      | % Get user-defined parameters
      | par.init_SOC   = init_SOC;
  EL0004_buckCCM : Subsystem  mask{R=1e-3, C=1, L=1e-6, V_init=400}
      mask prompts: R "Resistance [Ohm]:"; C "Capacity [F]:"; L "Inductance [H]:"; V_init "Voltage initial condition [V]:"
  EL0005_boostCCM : Subsystem  mask{C=1, L=1, eta=0.9, V_init=420}
      mask prompts: C "Capacity [F]:"; L "Inductance [H]:"; eta "Efficiency [-]:"; V_init "Voltage initial condition [V]:"
  EL0006_busDC : Subsystem  mask{R=1e-3, C=1, L=912e-9, V_init=420}
      mask prompts: R "Resistance [Ohm]:"; C "Capacitance [F]:"; L "Inductance [H]:"; V_init "Voltage initial condition [V]:"
  EL0007_pukrushpan2004 : Subsystem  mask{U_0=1, j_0=1e-3, alpha=0.25, ASR=1e-1, A_fc=300}
      mask prompts: U_0 "Open circuit voltage [V]:"; j_0 "Exchange current density [A/cm2]:"; alpha "Act. bar. symmetry [-]:"; ASR "Area specific resistance [ohm*cm2]:"; A_fc "Membrane area [cm2]:"
      mask init:
      | % parameter struct
      | par = struct;
      | 
      | % Get user-defined parameters
      | par.j_0   = j_0;
      | par.alpha = alpha;
      | par.ASR   = ASR;
      | par.U_0   = U_0;
      | par.A_fc  = A_fc;
      | 
      | % membrane thickness
      | par.t_m    = 0.01275;
      | 
      | % Molar mass - [kg/mol]
      | par.M_j  = [0.002;
      |             0.032;
      |             0.018;
      |             0.028];    
      | 
      | % Specific heat - [J/kg*K]        
      | par.cp_j = [14.43e3;
      |             0.928e3;
      |             1.996e3;
      |             1.041e3];  
      | 
      | % Universal gas constant - [J/(mol*K)]   
      | par.R  = 8.314;         
      | 
      | % Specific gas constant [J/kg*K]
      | par.R_j = par.R ./ par.M_j;
  EL0008_dcdcConverter : Subsystem  mask{eta_up=0.99, eta_down=0.99}
      mask prompts: eta_up "Efficiency up [-]"; eta_down "Efficiency down [-]"
      mask init:
      | par = struct;
      | par.eta_up = eta_up;
      | par.eta_down = eta_down;
  EL0010_superCapacitor : Subsystem  mask{C=1, V_bus0=700}
      mask prompts: C "Capacity [F]:"; V_bus0 "Initial voltage [V]:"
  EL0011_ITPEMFC : Subsystem  mask{A_fc=300}
      mask prompts: A_fc "Membrane area [cm2]:"
      mask init:
      | % parameter struct
      | par = struct;
      | 
      | % parameters
      | par.x = [0.375708611650636;
      |         -7.99625852105523e-07;
      |     	-1.12956449133080e-12;
      |     	0;
      |     	-2.75385376771518e-07;
      |     	0; 0;
      |     	58.0545571761230;
      |     	0; 0; 0; 0;	
      |         0.000242029125210931;
      |     	0;	0;	0;	0;	0;
      |     	0.0343867174128148;
      |     	0;
      |     	-7.27344985921884e-07;
      |     	0;
      |     	0.101451431061965;
      |     	0;	
      |         0;	
      |         96418140.2167285;	
      |         0;
      |     	5899.42812536311];
      | 
      | % Area
      | par.A_fc = A_fc;
      | 
      | 
      | % Molar mass - [kg/mol]
      | par.M_j  = [0.002;
      |             0.032;
      |             0.018;
      |             0.028];    
      | 
      | % Specific heat - [J/kg*K]        
      | par.cp_j = [14.43e3;
      |             0.928e3;
      |             1.996e3;
      |             1.041e3];  
      | 
      | % Universal gas constant - [J/(mol*K)]   
      | par.R  = 8.314;         
      | 
      | % Specific gas constant [J/kg*K]
      | par.R_j = par.R ./ par.M_j;

== system component_lib/Fuel Cell System ==
  I [A] : Inport
  throttle [-] : Inport  Port=2
  w_cmp [rad/s] : Inport  Port=3
  W_H2_ref [kg/s] : Inport  Port=4
  amb (T,p,RH) : Inport  Port=5
  T [K] : Inport  Port=6
  Anode Gas Exchange : $bdroot/Anode Gas Exchange  SystemSampleTime=-1  VariantActivationTime=update diagram  Latency=0  AutoFrameSizeCalculation=off
  Cathode Gas Exchange : $bdroot/Cathode Gas Exchange  SystemSampleTime=-1  VariantActivationTime=update diagram  Latency=0  AutoFrameSizeCalculation=off
  Constant4 : Constant  Value=n
  EL0007_pukrushpan2004 : $bdroot/Electrochemistry/EL0007_pukrushpan2004  U_0=1  j_0=1e-3  alpha=0.25  ASR=1e-1  A_fc=420
  F0010_vaporSaturationPressure.m : base_lib/F0010_gasFlow/F0010_vaporSaturationPressure.m  SystemSampleTime=-1  VariantActivationTime=update diagram  Latency=0  AutoFrameSizeCalculation=off
      settings: LibrarySourceBlock=|
      | simulink/User-Defined
      | Functions/MATLAB Function
  Gain{,1..3} (4 alike) : Gain  Gain=n_st
  Gain4 : Gain  Gain=1/420
  Product{1..5} (5 alike) : Product
  SC0002_signalRead1 : $bdroot/Data & Control/SC0002_signalRead  SigName=fuelCellVoltage
  SC0002_signalRead2 : $bdroot/Data & Control/SC0002_signalRead  SigName=fuelCellCurrent
  SC0002_signalRead3 : $bdroot/Data & Control/SC0002_signalRead  SigName=membraneWaterContent
  SC0002_signalRead4 : $bdroot/Data & Control/SC0002_signalRead  SigName=fuelCellPower
  SC0002_signalRead5 : $bdroot/Data & Control/SC0002_signalRead  SigName=vaporSaturationPressure
  SC0002_signalRead6 : $bdroot/Data & Control/SC0002_signalRead  SigName=singleCellVoltage
  SC0002_signalRead7 : $bdroot/Data & Control/SC0002_signalRead  SigName=compressorPower
  SC0002_signalRead8 : $bdroot/Data & Control/SC0002_signalRead  SigName=currentDensity
  Subsystem1 : Subsystem
      mask Display: disp('Fuel consumption calculation [kg/100km]');
  V [V] : Outport
  Q_gen [J/s] : Outport  Port=2
  P_cmp [J/s] : Outport  Port=3
  wires:
  Product1/1 -> Gain1/1
  EL0007_pukrushpan2004/1 -> Product1/1, SC0002_signalRead6/1
  Product2/1 -> [W_an], Gain/1
  Product5/1 -> [W_ca]
  Constant4/1 -> Product1/2, Product2/2, Product5/2, Product3/2
  I [A]/1 -> EL0007_pukrushpan2004/1, SC0002_signalRead2/1, Product4/1, Gain4/1
  EL0007_pukrushpan2004/3 -> Product5/1
  EL0007_pukrushpan2004/2 -> Product2/1
  EL0007_pukrushpan2004/5 -> Product3/1
  Product4/1 -> SC0002_signalRead4/1
  EL0007_pukrushpan2004/4 -> SC0002_signalRead3/1
  T [K]/1 -> F0010_vaporSaturationPressure.m/1, Anode Gas Exchange/3, Cathode Gas Exchange/5, EL0007_pukrushpan2004/4, EL0007_pukrushpan2004/5, EL0007_pukrushpan2004/6
  Cathode Gas Exchange/2 -> Gain3/1
  amb (T,p,RH)/1 -> Cathode Gas Exchange/4
  F0010_vaporSaturationPressure.m/1 -> SC0002_signalRead5/1
  Cathode Gas Exchange/1 -> EL0007_pukrushpan2004/3
  [W_ca] -> Cathode Gas Exchange/1
  Gain3/1 -> SC0002_signalRead7/1, P_cmp [J/s]/1
  Gain/1 -> Subsystem1/1(In1)
  Gain1/1 -> V [V]/1, SC0002_signalRead1/1, Product4/2
  Product3/1 -> Gain2/1
  Gain2/1 -> Q_gen [J/s]/1
  throttle [-]/1 -> Cathode Gas Exchange/2
  w_cmp [rad/s]/1 -> Cathode Gas Exchange/3
  Anode Gas Exchange/1 -> EL0007_pukrushpan2004/2
  [W_an] -> Anode Gas Exchange/1
  Gain4/1 -> SC0002_signalRead8/1
  W_H2_ref [kg/s]/1 -> Anode Gas Exchange/2
